simulink model "Template_v4_1_0_2024b_Jetson"  (R2024b)
settings: Solver=ode4  StartTime=0.0  StopTime=tsim  FixedStep=baseRate  RelTol=1e-6  AbsTol=1e-6
undefined symbols (not defined in the file): a1, a2, a3, b0, b1, b2, b3, baseRate, dataRate, DiscIntNeverNeededParam, drop_states_ARM, drop_states_BLACK, drop_states_BLUE, drop_states_RED, F_black_X_nominal, F_black_Y_nominal, F_blue_X_nominal, F_blue_Y_nominal, F_red_X_nominal, F_red_Y_nominal, F_thrusters_BLACK, F_thrusters_BLUE, F_thrusters_RED, Gamma1_el, Gamma1_sh, Gamma1_wr, Gamma2_el, Gamma2_sh, Gamma2_wr, Gamma3_el, Gamma3_sh, Gamma3_wr, Gamma4_el, Gamma4_sh, Gamma4_wr, Gamma5_el, Gamma5_sh, Gamma5_wr, Gamma6_el, Gamma6_sh, Gamma6_wr, home_states_BLACK, home_states_BLUE, home_states_RED, IBLACK, IBLUE, IDIST, IEE, init_states_BLACK, init_states_BLUE, init_states_RED, IPROX, IRED, K_BLACK, K_BLUE, K_RED, Kd_elarm, Kd_sharm, Kd_tb, Kd_tblue ... (+49)
libraries: simulink x30, dspsigops x12, nvidiaSharedBlocks x12, MainLibrary x5, dspinverses x3, nvidiaIMUSensorslib x1
(part 3 of 7)

== system Template_v4_1_0_2024b_Jetson/Gyro.//Accel. Code/Log Gyro//Accel ==
  Action Port : ActionPort  ActionPortLabel=if(u1 == 0)
  Data Store Read : DataStoreRead  DataStoreName=WhoAmI  IndexOptions=Index vector (dialog)  Indices=1  OutputSizes=1
  Data Store Write10 : DataStoreWrite  DataStoreName=BLACK_IMU_Measurements  IndexOptions=Index vector (dialog)  Indices=1  OutputSizes=1
  Data Store Write11 : DataStoreWrite  DataStoreName=BLUE_IMU_Measurements  IndexOptions=Index vector (dialog)  Indices=1  OutputSizes=1
  Data Store Write9 : DataStoreWrite  DataStoreName=RED_IMU_Measurements  IndexOptions=Index vector (dialog)  Indices=1  OutputSizes=1
  Demux : Demux  Outputs=3
  Demux1 : Demux  Outputs=3
  Gyroscope/Accelerometer : nvidiaIMUSensorslib/BMI160  I2CModule=1  I2CAddress=0x69  EnableSecondaryMag=on  MagnetometerI2CAddress=0x10  BitRate=1000000  IsActiveAccel=on  IsActiveGyro=on  IsActiveMag=off  IsActiveTemperature=off  IsIntSource=off  IsTapEventSource=off  IsHighGEventSource=off  IsAnyMotionEventSource=off  IsAccelStatus=off  IsGyroStatus=off  IsMagStatus=off  AccelerationRange=+/- 2g  AccelerometerODR=100 Hz  IsEnableAccelLowPassFilter=off  AccelerometerFilterMode=Normal  GyroscopeRange=125 dps  GyroscopeODR=100 Hz  IsEnableGyroLowPassFilter=off  GyroscopeFilterMode=Normal  MagnetometerODR=25 Hz  IsSingleTap=off  SingleTapQuietTimeThreshold=30 ms  SingleTapShockTimeThreshold=50 ms  SingleTapAmplitudeThreshold2g=0.1  SingleTapAmplitudeThreshold4g=0.1  SingleTapAmplitudeThreshold8g=0.2  SingleTapAmplitudeThreshold16g=0.3  InterruptPinSingleTap=INT1  IsDoubleTap=off  DoubleTapDurationTimeThreshold=50 ms  InterruptPinDoubleTap=INT1  IsHighGDetection=off  HighGTimeThreshold=2.5  HighGAmplitudeThreshold2g=0.1  HighGAmplitudeThreshold4g=0.1  HighGAmplitudeThreshold8g=0.1  HighGAmplitudeThreshold16g=0.1  InterruptPinHighG=INT1  IsAnyMotion=off  AnyMotionTimeThreshold=1  AnyMotionAmplitudeThreshold2g=0.1  AnyMotionAmplitudeThreshold4g=0.1  AnyMotionAmplitudeThreshold8g=0.1  AnyMotionAmplitudeThreshold16g=0.1  InterruptPinAnyMotion=INT1  IsSlowMotion=off  SlowMotionTimeThreshold=1  SlowMotionAmplitudeThreshold2g=0.1  SlowMotionAmplitudeThreshold4g=0.1  SlowMotionAmplitudeThreshold8g=0.1  SlowMotionAmplitudeThreshold16g=0.1  InterruptPinSlowMotion=INT1  IsFlatDetection=off  FlatThetaThreshold=5  FlatTimeThreshold=640 ms  InterruptPinFlat=INT1  IsDataReady=off  InterruptPinDataReady=INT1  IsFifo=off  FifoMode=Full Buffer  InterruptPinFifo=INT1  DataType=double  SampleTime=-1
  Mux : Mux  Inputs=3
  Mux1 : Mux  Inputs=3
  Mux2 : Mux  Inputs=3
  Parse IMU Data : MATLAB Function  TreatAsAtomicUnit=on
  Terminator : Terminator
  Terminator1 : Terminator
  Terminator2 : Terminator
  wires:
  Demux1/3 -> Parse IMU Data/4(IMU_Gz)
  Gyroscope/Accelerometer/1 -> Demux/1
  Demux1/1 -> Terminator1/1
  Parse IMU Data/4(BLACK_IMU_Ax) -> Mux1/1
  Parse IMU Data/1(RED_IMU_Ax) -> Mux/1
  Parse IMU Data/8(BLUE_IMU_Ay) -> Mux2/2
  Parse IMU Data/3(RED_IMU_Gz) -> Mux/3
  Demux/3 -> Terminator/1
  Parse IMU Data/6(BLACK_IMU_Gz) -> Mux1/3
  Parse IMU Data/5(BLACK_IMU_Ay) -> Mux1/2
  Demux1/2 -> Terminator2/1
  Parse IMU Data/9(BLUE_IMU_Gz) -> Mux2/3
  Gyroscope/Accelerometer/2 -> Demux1/1
  Parse IMU Data/2(RED_IMU_Ay) -> Mux/2
  Parse IMU Data/7(BLUE_IMU_Ax) -> Mux2/1
  Demux/2 -> Parse IMU Data/3(IMU_Ay)
  Data Store Read/1 -> Parse IMU Data/1(WhoAmI)
  Demux/1 -> Parse IMU Data/2(IMU_Ax)
  Mux/1 -> Data Store Write9/1
  Mux1/1 -> Data Store Write10/1
  Mux2/1 -> Data Store Write11/1

== system Template_v4_1_0_2024b_Jetson/Manipulator Encoder Data/Change ARM Behavior ==
  Action Port : ActionPort  ActionPortLabel=if(u1 == 1 & u2 == 0)
  Data Store Write : DataStoreWrite  DataStoreName=ARM_Measured_States  IndexOptions=Index vector (dialog)  Indices=1  OutputSizes=1
  Delay : Delay  DelayLength=1
  Delay1 : Delay  DelayLength=1
  Delay2 : Delay  DelayLength=1
  Mux : Mux  Inputs=6
  Read Joint Positions using Dynamixel Encoders : MainLibrary/Dynamixel Functions/Read Joint Positions using  Dynamixel Encoders  SampleTime=baseRate
      settings: SourceProductName=SPOT Custom Library
  wires:
  Delay/1 -> Read Joint Positions using Dynamixel Encoders/1
  Read Joint Positions using Dynamixel Encoders/5 -> Mux/5
  Read Joint Positions using Dynamixel Encoders/6 -> Mux/6
  Delay1/1 -> Read Joint Positions using Dynamixel Encoders/2
  Read Joint Positions using Dynamixel Encoders/2 -> Mux/2, Delay1/1
  Delay2/1 -> Read Joint Positions using Dynamixel Encoders/3
  Read Joint Positions using Dynamixel Encoders/1 -> Mux/1, Delay/1
  Read Joint Positions using Dynamixel Encoders/3 -> Mux/3, Delay2/1
  Read Joint Positions using Dynamixel Encoders/4 -> Mux/4
  Mux/1 -> Data Store Write/1

== system Template_v4_1_0_2024b_Jetson/PhaseSpace Camera Code/Initialize Universal Time (Simulation) ==
  Action Port : ActionPort  ActionPortLabel=elseif(u1 == 1)
  Set Universal Time (If this is a simulation) : Clock
  Universal_Time : DataStoreWrite  DataStoreName=Univ_Time  IndexOptions=Index vector (dialog)  Indices=1  OutputSizes=1
  wires:
  Set Universal Time (If this is a simulation)/1 -> Universal_Time/1

== system Template_v4_1_0_2024b_Jetson/PhaseSpace Camera Code/Use Hardware to Obtain States ==
  Action Port : ActionPort  ActionPortLabel=if(u1 == 0)
  Demux : Demux  Outputs=[4,3,3,9]
  Demux1 : Demux  Outputs=[3,3,3]
  Receive and Process Phasespace Data : Subsystem
  Store BLACK Data : Subsystem
  Store BLUE Data : Subsystem
  Store RED Data : Subsystem
  wires:
  Receive and Process Phasespace Data/1(PhaseSpace Data) -> Demux/1
  Demux/1 -> Store RED Data/1(RED Data)
  Demux/2 -> Store BLACK Data/1(BLACK Data)
  Demux/3 -> Store BLUE Data/1(BLUE Data)
  Demux/4 -> Demux1/1
  Demux1/1 -> Store RED Data/2(RED Velocities)
  Demux1/2 -> Store BLACK Data/2(BLACK Velocities)
  Demux1/3 -> Store BLUE Data/2(BLUE Velocities)
  Receive and Process Phasespace Data/2(PhaseSpace Clock) -> Store RED Data/3(PS Clock), Store BLACK Data/3(PS Clock), Store BLUE Data/3(PS Clock)

== system Template_v4_1_0_2024b_Jetson/Platform Identification/Subsystem ==
  Action Port : ActionPort  ActionPortLabel=if(u1 == 0)
  Data Store Write : DataStoreWrite  DataStoreName=WhoAmI  IndexOptions=Index vector (dialog)  Indices=1  OutputSizes=1
  WhoAmI : MainLibrary/WhoAmI  SampleTime=baseRate
      settings: SourceProductName=SPOT Custom Library
  wires:
  WhoAmI/1 -> Data Store Write/1

== system Template_v4_1_0_2024b_Jetson/Robotic Arm Code/Change ARM Behavior ==
  Action Port : ActionPort  ActionPortLabel=if(u1 == 1 & u2 == 0)
  Arm Control Mode : DataStoreRead  DataStoreName=ARM_Control_Mode  IndexOptions=Index vector (dialog)  Indices=1  OutputSizes=1
  Command : DataStoreRead  DataStoreName=ARM_Controls  IndexOptions=Index vector (dialog)  Indices=1  OutputSizes=1
  "Control Dynamixel Actuators in either Position, Current, or Speed Control Modes" : MainLibrary/Dynamixel Functions/Control Dynamixel Actuators in  either Position, Current, or Speed  Control Modes  POSITION_P_GAIN=400  POSITION_I_GAIN=0  POSITION_D_GAIN=200  MAX_POSITION=3072  MIN_POSITION=1024  MOVE_TIME=0  CURRENT_LIMIT=850  SPEED_P_GAIN=400  SPEED_I_GAIN=100  VELOCITY_LIMIT=50  ACCELERATION_TIME=0  SampleTime=baseRate
      settings: SourceProductName=SPOT Custom Library
  Demux : Demux  Outputs=3
  wires:
  Arm Control Mode/1 -> "Control Dynamixel Actuators in either Position, Current, or Speed Control Modes"/1
  Command/1 -> Demux/1
  Demux/1 -> "Control Dynamixel Actuators in either Position, Current, or Speed Control Modes"/2
  Demux/2 -> "Control Dynamixel Actuators in either Position, Current, or Speed Control Modes"/3
  Demux/3 -> "Control Dynamixel Actuators in either Position, Current, or Speed Control Modes"/4

== system Template_v4_1_0_2024b_Jetson/Send Data to Orin/Subsystem ==
  Action Port : ActionPort  ActionPortLabel=if(u1 == 0)
  BLACK States : DataStoreRead  DataStoreName=BLACK_Measured_States  IndexOptions=Index vector (dialog)  Indices=1  OutputSizes=1
  BLUE States : DataStoreRead  DataStoreName=BLUE_Measured_States  IndexOptions=Index vector (dialog)  Indices=1  OutputSizes=1
  Mux : Mux
  RED States : DataStoreRead  DataStoreName=RED_Measured_States  IndexOptions=Index vector (dialog)  Indices=1  OutputSizes=1
  Time : DataStoreRead  DataStoreName=Univ_Time  IndexOptions=Index vector (dialog)  Indices=1  OutputSizes=1
  UDP Send : nvidiaSharedBlocks/UDP Send  remoteURL='192.168.1.115'  remotePort=46875  localURL='0.0.0.0'  localPortSource=Automatically determine  localPort=-1  sampletime=-1  blockPlatform=NVIDIA  separateLengthPort=0
      settings: LibrarySourceBlock=nvidiaNetworklib/UDP Send
  wires:
  Mux/1 -> UDP Send/1
  Time/1 -> Mux/1
  RED States/1 -> Mux/2
  BLACK States/1 -> Mux/3
  BLUE States/1 -> Mux/4

== system Template_v4_1_0_2024b_Jetson/Simulate Plant Dynamics/BLACK Dynamics ==
  Add Noise : RandomNumber  Variance=1e-9  SampleTime=baseRate
  Calculated & Store Measured States : Subsystem
  Calculated & Store True States : Subsystem
  Data @ Measurement Rate : Subsystem
  Dynamics Model for BLACK : Subsystem  SystemSampleTime=serverRate
      settings: PortSchema="{\"entries\":[{\"content\":{\"sides\":[{\"content\":{\"connectorIds\":[\"In1\"]},\"type\":\"ConnectorPlacement.EquallySpacedRectSide\",\"uuid\":\"9df3cfb7-f920-4c45-b004-2d63eab5f007\"},{\"content\":{\"side\":\"RIGHT\"},\"type\":\"ConnectorPlacement.EquallySpacedRectSide\",\"uuid\":\"24f4b70f-864f-4cab-bc2b-b450467a01b3\"},{\"content\":{\"connectorIds\":[\"Out1\"],\"side\":\"TOP\"},\"type\":\"ConnectorPlacement.EquallySpacedRectSide\",\"uuid\":\"64c0236c-f70a-4099-950e-ee3e8643e7f2\"}]},\"type\":\"ConnectorPlacement.EquallySpacedConnector\",\"uuid\":\"dd7c693a-185b-4c5f-873e-b9df56bea395\"}],\"packageUris\":[\"http://schema.mathworks.com/mf0/Connector/R2020b\"],\"version\":\"1.0\"}"
  Saturated Control Commands for BLACK : DataStoreRead  DataStoreName=BLACK_Saturated_Controls  IndexOptions=Index vector (dialog)  Indices=1  OutputSizes=1
  Sum : Sum  Inputs=++|
  wires:
  Dynamics Model for BLACK/1(states) -> Sum/2, Calculated & Store True States/1(y)
  Data @ Measurement Rate/2(Time Step) -> Calculated & Store Measured States/2(dt)
  Saturated Control Commands for BLACK/1 -> Dynamics Model for BLACK/1(control_inputs)
  Data @ Measurement Rate/1(Data Held) -> Calculated & Store Measured States/1(y)
  Sum/1 -> Data @ Measurement Rate/1(Data Input)
  Add Noise/1 -> Sum/1

== system Template_v4_1_0_2024b_Jetson/Simulate Plant Dynamics/BLUE Dynamics ==
  Add Noise : RandomNumber  Variance=1e-9  SampleTime=baseRate
  BLUE  Dynamics Model : Subsystem  SystemSampleTime=serverRate
      settings: PortSchema="{\"entries\":[{\"content\":{\"sides\":[{\"content\":{\"connectorIds\":[\"In1\"]},\"type\":\"ConnectorPlacement.EquallySpacedRectSide\",\"uuid\":\"9df3cfb7-f920-4c45-b004-2d63eab5f007\"},{\"content\":{\"side\":\"RIGHT\"},\"type\":\"ConnectorPlacement.EquallySpacedRectSide\",\"uuid\":\"24f4b70f-864f-4cab-bc2b-b450467a01b3\"},{\"content\":{\"connectorIds\":[\"Out1\"],\"side\":\"TOP\"},\"type\":\"ConnectorPlacement.EquallySpacedRectSide\",\"uuid\":\"64c0236c-f70a-4099-950e-ee3e8643e7f2\"}]},\"type\":\"ConnectorPlacement.EquallySpacedConnector\",\"uuid\":\"dd7c693a-185b-4c5f-873e-b9df56bea395\"}],\"packageUris\":[\"http://schema.mathworks.com/mf0/Connector/R2020b\"],\"version\":\"1.0\"}"
  Calculated & Store Measured States : Subsystem
  Calculated & Store True States : Subsystem
  Data @ Measurement Rate : Subsystem
  Saturated Control Commands for BLUE : DataStoreRead  DataStoreName=BLUE_Saturated_Controls  IndexOptions=Index vector (dialog)  Indices=1  OutputSizes=1
  Sum1 : Sum  Inputs=++|
  wires:
  Saturated Control Commands for BLUE/1 -> BLUE  Dynamics Model/1(control_inputs)
  Data @ Measurement Rate/2(Time Step) -> Calculated & Store Measured States/2(dt)
  Add Noise/1 -> Sum1/1
  BLUE  Dynamics Model/1(states) -> Sum1/2, Calculated & Store True States/1(y)
  Sum1/1 -> Data @ Measurement Rate/1(Data Input)
  Data @ Measurement Rate/1(Data Held) -> Calculated & Store Measured States/1(y)

== system Template_v4_1_0_2024b_Jetson/Simulate Plant Dynamics/RED and ARM Dynamics ==
  Constant : Constant  Value=platformSelection
  If : If  IfExpression=u1 == 4 | u1 == 5 | u1 == 10 | u1 == 11
  RED + ARM : Subsystem  TreatAsAtomicUnit=on
  RED Only : Subsystem  TreatAsAtomicUnit=on
  wires:
  If/1 -> RED + ARM/Action
  Constant/1 -> If/1
  If/2 -> RED Only/Action

== system Template_v4_1_0_2024b_Jetson/Thruster Control Code/Change BLACK Behavior ==
  note: Calculate the percentage of time each thruster must be on, and send to the PWM blocks.
  note: Using the attitude, rotate the forces into the body frame.
  note: Calculate which thrusters must be turned on and for how long.
  Action Port : ActionPort  ActionPortLabel=if(u1 == 2 | u2 == 1)
  BLACK Controls : DataStoreRead  DataStoreName=BLACK_Controls  IndexOptions=Index vector (dialog)  Indices=1  OutputSizes=1
  BLACK States : DataStoreRead  DataStoreName=BLACK_Measured_States  IndexOptions=Index vector (dialog)  Indices=1  OutputSizes=1
  Calculate Duty Cycle : Subsystem
  Data Store Write2 : DataStoreWrite  DataStoreName=BLACK_Saturated_Controls  IndexOptions=Index vector (dialog)  Indices=1  OutputSizes=1
  Demux1 : Demux  Outputs=[2,1]
  Demux2 : Demux  Outputs=[2,1,6]
  Mux : Mux  Inputs=2
  Rotate Forces to Body : Subsystem
  Terminator : Terminator
  Terminator1 : Terminator
  BLACK DC : Outport  VectorParamsAs1DForOutWhenUnconnected=off
  wires:
  Calculate Duty Cycle/2(Saturated Forces Moments) -> Data Store Write2/1
  Rotate Forces to Body/1(F_b) -> Mux/1
  Demux1/2 -> Mux/2
  Calculate Duty Cycle/1(Duty Cycle) -> BLACK DC/1
  Mux/1 -> Calculate Duty Cycle/1("[Fx_b; Fy_b; Tz]")
  BLACK Controls/1 -> Demux1/1
  Demux1/1 -> Rotate Forces to Body/1("F_I ")
  BLACK States/1 -> Demux2/1
  Demux2/1 -> Terminator/1
  Demux2/3 -> Terminator1/1
  Demux2/2 -> Calculate Duty Cycle/2(Measured Attitude), Rotate Forces to Body/2(Rz)

== system Template_v4_1_0_2024b_Jetson/Thruster Control Code/Change BLUE Behavior ==
  note: Calculate the percentage of time each thruster must be on, and send to the PWM blocks.
  note: Using the attitude, rotate the forces into the body frame.
  note: Calculate which thrusters must be turned on and for how long.
  Action Port : ActionPort  ActionPortLabel=if(u1 == 3 | u2 == 1)
  Calculate Duty Cycle : Subsystem
  Data Store Read : DataStoreRead  DataStoreName=BLUE_Controls  IndexOptions=Index vector (dialog)  Indices=1  OutputSizes=1
  Data Store Read1 : DataStoreRead  DataStoreName=BLUE_Measured_States  IndexOptions=Index vector (dialog)  Indices=1  OutputSizes=1
  Data Store Write3 : DataStoreWrite  DataStoreName=BLUE_Saturated_Controls  IndexOptions=Index vector (dialog)  Indices=1  OutputSizes=1
  Demux : Demux  Outputs=[2,1]
  Demux1 : Demux  Outputs=[2,1,6]
  Mux1 : Mux  Inputs=2
  Rotate Forces to Body : Subsystem
  Terminator : Terminator
  Terminator1 : Terminator
  BLUE DC : Outport  VectorParamsAs1DForOutWhenUnconnected=off
  wires:
  Calculate Duty Cycle/1(Duty Cycle) -> BLUE DC/1
  Rotate Forces to Body/1(F_b) -> Mux1/1
  Demux/2 -> Mux1/2
  Mux1/1 -> Calculate Duty Cycle/1("[Fx_b; Fy_b; Tz]")
  Calculate Duty Cycle/2(Saturated Forces Moments) -> Data Store Write3/1
  Data Store Read/1 -> Demux/1
  Demux/1 -> Rotate Forces to Body/1("F_I ")
  Data Store Read1/1 -> Demux1/1
  Demux1/2 -> Calculate Duty Cycle/2(Measured Attitude), Rotate Forces to Body/2(Rz)
  Demux1/1 -> Terminator/1
  Demux1/3 -> Terminator1/1

== system Template_v4_1_0_2024b_Jetson/Thruster Control Code/Change RED Behavior ==
  note: Calculate which thrusters must be turned on and for how long.
  note: Calculate the percentage of time each thruster must be on, and send to the PWM blocks.
  note: Using the attitude, rotate the forces into the body frame.
  Action Port : ActionPort  ActionPortLabel=if(u1 == 1 | u2 == 1)
  Calculate Duty Cycle : Subsystem
  Data Store Read : DataStoreRead  DataStoreName=RED_Controls  IndexOptions=Index vector (dialog)  Indices=1  OutputSizes=1
  Data Store Read1 : DataStoreRead  DataStoreName=RED_Measured_States  IndexOptions=Index vector (dialog)  Indices=1  OutputSizes=1
  Data Store Write3 : DataStoreWrite  DataStoreName=RED_Saturated_Controls  IndexOptions=Index vector (dialog)  Indices=1  OutputSizes=1
  Demux : Demux  Outputs=[2,1]
  Demux1 : Demux  Outputs=[2,1,6]
  Mux1 : Mux  Inputs=2
  Rotate Forces to Body : Subsystem
  Terminator : Terminator
  Terminator1 : Terminator
  RED DC : Outport  VectorParamsAs1DForOutWhenUnconnected=off
  wires:
  Calculate Duty Cycle/2(Saturated Forces Moments) -> Data Store Write3/1
  Demux/1 -> Rotate Forces to Body/1("F_I ")
  Mux1/1 -> Calculate Duty Cycle/1("[Fx_b; Fy_b; Tz]")
  Demux/2 -> Mux1/2
  Demux1/2 -> Calculate Duty Cycle/2(Measured Attitude), Rotate Forces to Body/2(Rz)
  Rotate Forces to Body/1(F_b) -> Mux1/1
  Calculate Duty Cycle/1(Duty Cycle) -> RED DC/1
  Data Store Read/1 -> Demux/1
  Demux1/1 -> Terminator/1
  Demux1/3 -> Terminator1/1
  Data Store Read1/1 -> Demux1/1

== system Template_v4_1_0_2024b_Jetson/1 - Experiment Logic/Phase #2: Initial Position/Desired Joint Angles RED ==
  Constant1 : Constant  Value=pi/2
  Constant2 : Constant  Value=0
  Constant3 : Constant  Value=pi/2
  Mux : Mux  Inputs=3
  Target Array : Outport
  wires:
  Mux/1 -> Target Array/1
  Constant3/1 -> Mux/1
  Constant1/1 -> Mux/2
  Constant2/1 -> Mux/3

== system Template_v4_1_0_2024b_Jetson/1 - Experiment Logic/Phase #2: Initial Position/Desired Position BLACK ==
  Desired States (BLACK) : Constant  Value=init_states_BLACK  SampleTime=-1
  Target Array : Outport
  wires:
  Desired States (BLACK)/1 -> Target Array/1

== system Template_v4_1_0_2024b_Jetson/1 - Experiment Logic/Phase #2: Initial Position/Desired Position BLUE ==
  Desired States (BLUE) : Constant  Value=init_states_BLUE  SampleTime=-1
  Target Array : Outport
  wires:
  Desired States (BLUE)/1 -> Target Array/1

== system Template_v4_1_0_2024b_Jetson/1 - Experiment Logic/Phase #2: Initial Position/Desired Position RED ==
  Constant2 : Constant  Value=init_states_RED
  Target Array : Outport
  wires:
  Constant2/1 -> Target Array/1

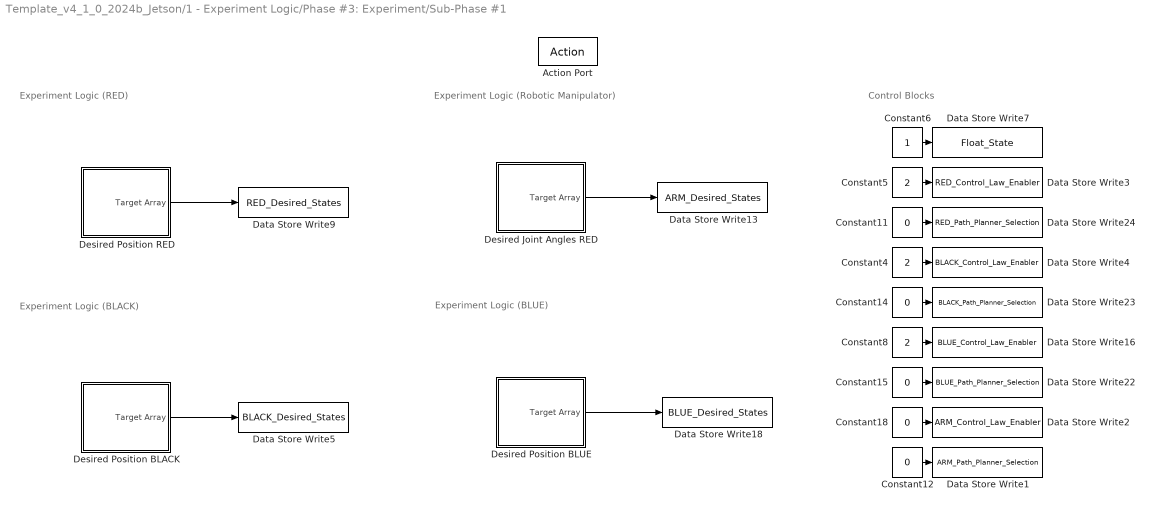
== system Template_v4_1_0_2024b_Jetson/1 - Experiment Logic/Phase #3: Experiment/Sub-Phase #1 ==
  note: Experiment Logic (BLUE)
  note: Experiment Logic (Robotic Manipulator)
  note: Experiment Logic (RED)
  note: Experiment Logic (BLACK)
  note: Control Blocks
  Action Port : ActionPort  ActionPortLabel=if(u1 < u2)
  Constant{11..12,14..15,18} (5 alike) : Constant  Value=0
  Constant4 : Constant  Value=2
  Constant5 : Constant  Value=2
  Constant6 : Constant
  Constant8 : Constant  Value=2
  Data Store Write1 : DataStoreWrite  DataStoreName=ARM_Path_Planner_Selection  IndexOptions=Index vector (dialog)  Indices=1  OutputSizes=1
  Data Store Write13 : DataStoreWrite  DataStoreName=ARM_Desired_States  IndexOptions=Index vector (dialog)  Indices=1  OutputSizes=1
  Data Store Write16 : DataStoreWrite  DataStoreName=BLUE_Control_Law_Enabler  IndexOptions=Index vector (dialog)  Indices=1  OutputSizes=1
  Data Store Write18 : DataStoreWrite  DataStoreName=BLUE_Desired_States  IndexOptions=Index vector (dialog)  Indices=1  OutputSizes=1
  Data Store Write2 : DataStoreWrite  DataStoreName=ARM_Control_Law_Enabler  IndexOptions=Index vector (dialog)  Indices=1  OutputSizes=1
  Data Store Write22 : DataStoreWrite  DataStoreName=BLUE_Path_Planner_Selection  IndexOptions=Index vector (dialog)  Indices=1  OutputSizes=1
  Data Store Write23 : DataStoreWrite  DataStoreName=BLACK_Path_Planner_Selection  IndexOptions=Index vector (dialog)  Indices=1  OutputSizes=1
  Data Store Write24 : DataStoreWrite  DataStoreName=RED_Path_Planner_Selection  IndexOptions=Index vector (dialog)  Indices=1  OutputSizes=1
  Data Store Write3 : DataStoreWrite  DataStoreName=RED_Control_Law_Enabler  IndexOptions=Index vector (dialog)  Indices=1  OutputSizes=1
  Data Store Write4 : DataStoreWrite  DataStoreName=BLACK_Control_Law_Enabler  IndexOptions=Index vector (dialog)  Indices=1  OutputSizes=1
  Data Store Write5 : DataStoreWrite  DataStoreName=BLACK_Desired_States  IndexOptions=Index vector (dialog)  Indices=1  OutputSizes=1
  Data Store Write7 : DataStoreWrite  DataStoreName=Float_State  IndexOptions=Index vector (dialog)  Indices=1  OutputSizes=1
  Data Store Write9 : DataStoreWrite  DataStoreName=RED_Desired_States  IndexOptions=Index vector (dialog)  Indices=1  OutputSizes=1
  Desired Joint Angles RED : Subsystem
  Desired Position BLACK : Subsystem
  Desired Position BLUE : Subsystem
  Desired Position RED : Subsystem
  wires:
  Desired Position BLACK/1(Target Array) -> Data Store Write5/1
  Desired Position BLUE/1(Target Array) -> Data Store Write18/1
  Desired Position RED/1(Target Array) -> Data Store Write9/1
  Desired Joint Angles RED/1(Target Array) -> Data Store Write13/1
  Constant12/1 -> Data Store Write1/1
  Constant18/1 -> Data Store Write2/1
  Constant6/1 -> Data Store Write7/1
  Constant15/1 -> Data Store Write22/1
  Constant14/1 -> Data Store Write23/1
  Constant5/1 -> Data Store Write3/1
  Constant11/1 -> Data Store Write24/1
  Constant8/1 -> Data Store Write16/1
  Constant4/1 -> Data Store Write4/1

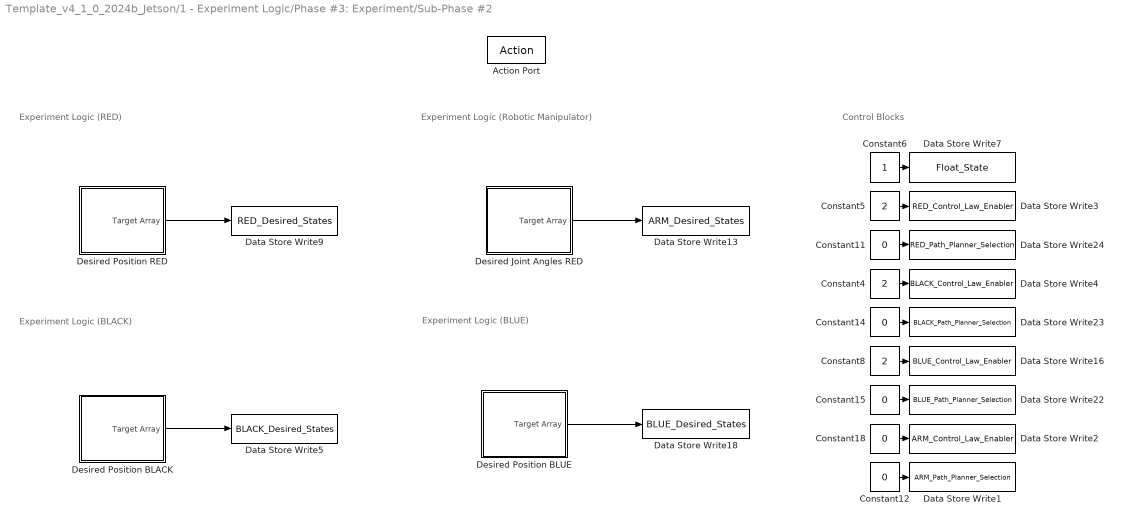
== system Template_v4_1_0_2024b_Jetson/1 - Experiment Logic/Phase #3: Experiment/Sub-Phase #2  ==
  note: Experiment Logic (BLACK)
  note: Experiment Logic (Robotic Manipulator)
  note: Experiment Logic (BLUE)
  note: Experiment Logic (RED)
  note: Control Blocks
  Action Port : ActionPort  ActionPortLabel=elseif((u1 < u3 & u1 >= u2))
  Constant{11..12,14..15,18} (5 alike) : Constant  Value=0
  Constant4 : Constant  Value=2
  Constant5 : Constant  Value=2
  Constant6 : Constant
  Constant8 : Constant  Value=2
  Data Store Write1 : DataStoreWrite  DataStoreName=ARM_Path_Planner_Selection  IndexOptions=Index vector (dialog)  Indices=1  OutputSizes=1
  Data Store Write13 : DataStoreWrite  DataStoreName=ARM_Desired_States  IndexOptions=Index vector (dialog)  Indices=1  OutputSizes=1
  Data Store Write16 : DataStoreWrite  DataStoreName=BLUE_Control_Law_Enabler  IndexOptions=Index vector (dialog)  Indices=1  OutputSizes=1
  Data Store Write18 : DataStoreWrite  DataStoreName=BLUE_Desired_States  IndexOptions=Index vector (dialog)  Indices=1  OutputSizes=1
  Data Store Write2 : DataStoreWrite  DataStoreName=ARM_Control_Law_Enabler  IndexOptions=Index vector (dialog)  Indices=1  OutputSizes=1
  Data Store Write22 : DataStoreWrite  DataStoreName=BLUE_Path_Planner_Selection  IndexOptions=Index vector (dialog)  Indices=1  OutputSizes=1
  Data Store Write23 : DataStoreWrite  DataStoreName=BLACK_Path_Planner_Selection  IndexOptions=Index vector (dialog)  Indices=1  OutputSizes=1
  Data Store Write24 : DataStoreWrite  DataStoreName=RED_Path_Planner_Selection  IndexOptions=Index vector (dialog)  Indices=1  OutputSizes=1
  Data Store Write3 : DataStoreWrite  DataStoreName=RED_Control_Law_Enabler  IndexOptions=Index vector (dialog)  Indices=1  OutputSizes=1
  Data Store Write4 : DataStoreWrite  DataStoreName=BLACK_Control_Law_Enabler  IndexOptions=Index vector (dialog)  Indices=1  OutputSizes=1
  Data Store Write5 : DataStoreWrite  DataStoreName=BLACK_Desired_States  IndexOptions=Index vector (dialog)  Indices=1  OutputSizes=1
  Data Store Write7 : DataStoreWrite  DataStoreName=Float_State  IndexOptions=Index vector (dialog)  Indices=1  OutputSizes=1
  Data Store Write9 : DataStoreWrite  DataStoreName=RED_Desired_States  IndexOptions=Index vector (dialog)  Indices=1  OutputSizes=1
  Desired Joint Angles RED : Subsystem
  Desired Position BLACK : Subsystem
  Desired Position BLUE : Subsystem
  Desired Position RED : Subsystem
  wires:
  Desired Position RED/1(Target Array) -> Data Store Write9/1
  Desired Position BLACK/1(Target Array) -> Data Store Write5/1
  Desired Position BLUE/1(Target Array) -> Data Store Write18/1
  Constant12/1 -> Data Store Write1/1
  Constant18/1 -> Data Store Write2/1
  Constant6/1 -> Data Store Write7/1
  Constant15/1 -> Data Store Write22/1
  Constant14/1 -> Data Store Write23/1
  Constant5/1 -> Data Store Write3/1
  Constant11/1 -> Data Store Write24/1
  Constant8/1 -> Data Store Write16/1
  Constant4/1 -> Data Store Write4/1
  Desired Joint Angles RED/1(Target Array) -> Data Store Write13/1

== system Template_v4_1_0_2024b_Jetson/1 - Experiment Logic/Phase #3: Experiment/Sub-Phase #3  ==
  note: Experiment Logic (BLACK)
  note: Experiment Logic (Robotic Manipulator)
  note: Experiment Logic (BLUE)
  note: Experiment Logic (RED)
  note: Control Blocks
  Action Port : ActionPort  ActionPortLabel=elseif((u1 < u4 & u1 >= u3))
  Constant{11..12,14..15,18} (5 alike) : Constant  Value=0
  Constant4 : Constant  Value=2
  Constant5 : Constant  Value=2
  Constant6 : Constant
  Constant8 : Constant  Value=2
  Data Store Write1 : DataStoreWrite  DataStoreName=ARM_Path_Planner_Selection  IndexOptions=Index vector (dialog)  Indices=1  OutputSizes=1
  Data Store Write13 : DataStoreWrite  DataStoreName=ARM_Desired_States  IndexOptions=Index vector (dialog)  Indices=1  OutputSizes=1
  Data Store Write16 : DataStoreWrite  DataStoreName=BLUE_Control_Law_Enabler  IndexOptions=Index vector (dialog)  Indices=1  OutputSizes=1
  Data Store Write18 : DataStoreWrite  DataStoreName=BLUE_Desired_States  IndexOptions=Index vector (dialog)  Indices=1  OutputSizes=1
  Data Store Write2 : DataStoreWrite  DataStoreName=ARM_Control_Law_Enabler  IndexOptions=Index vector (dialog)  Indices=1  OutputSizes=1
  Data Store Write22 : DataStoreWrite  DataStoreName=BLUE_Path_Planner_Selection  IndexOptions=Index vector (dialog)  Indices=1  OutputSizes=1
  Data Store Write23 : DataStoreWrite  DataStoreName=BLACK_Path_Planner_Selection  IndexOptions=Index vector (dialog)  Indices=1  OutputSizes=1
  Data Store Write24 : DataStoreWrite  DataStoreName=RED_Path_Planner_Selection  IndexOptions=Index vector (dialog)  Indices=1  OutputSizes=1
  Data Store Write3 : DataStoreWrite  DataStoreName=RED_Control_Law_Enabler  IndexOptions=Index vector (dialog)  Indices=1  OutputSizes=1
  Data Store Write4 : DataStoreWrite  DataStoreName=BLACK_Control_Law_Enabler  IndexOptions=Index vector (dialog)  Indices=1  OutputSizes=1
  Data Store Write5 : DataStoreWrite  DataStoreName=BLACK_Desired_States  IndexOptions=Index vector (dialog)  Indices=1  OutputSizes=1
  Data Store Write7 : DataStoreWrite  DataStoreName=Float_State  IndexOptions=Index vector (dialog)  Indices=1  OutputSizes=1
  Data Store Write9 : DataStoreWrite  DataStoreName=RED_Desired_States  IndexOptions=Index vector (dialog)  Indices=1  OutputSizes=1
  Desired Joint Angles RED : Subsystem
  Desired Position BLACK : Subsystem
  Desired Position BLUE : Subsystem
  Desired Position RED : Subsystem
  wires:
  Desired Position RED/1(Target Array) -> Data Store Write9/1
  Desired Position BLACK/1(Target Array) -> Data Store Write5/1
  Desired Position BLUE/1(Target Array) -> Data Store Write18/1
  Desired Joint Angles RED/1(Target Array) -> Data Store Write13/1
  Constant12/1 -> Data Store Write1/1
  Constant18/1 -> Data Store Write2/1
  Constant6/1 -> Data Store Write7/1
  Constant15/1 -> Data Store Write22/1
  Constant14/1 -> Data Store Write23/1
  Constant5/1 -> Data Store Write3/1
  Constant11/1 -> Data Store Write24/1
  Constant8/1 -> Data Store Write16/1
  Constant4/1 -> Data Store Write4/1

== system Template_v4_1_0_2024b_Jetson/1 - Experiment Logic/Phase #3: Experiment/Sub-Phase #4 ==
  note: Experiment Logic (BLACK)
  note: Experiment Logic (Robotic Manipulator)
  note: Experiment Logic (BLUE)
  note: Experiment Logic (RED)
  note: Control Blocks
  Action Port : ActionPort  ActionPortLabel=elseif( (u1 < u5 & u1 >= u4))
  Constant{11..12,14..15,18} (5 alike) : Constant  Value=0
  Constant4 : Constant  Value=2
  Constant5 : Constant  Value=2
  Constant6 : Constant
  Constant8 : Constant  Value=2
  Data Store Write1 : DataStoreWrite  DataStoreName=ARM_Path_Planner_Selection  IndexOptions=Index vector (dialog)  Indices=1  OutputSizes=1
  Data Store Write13 : DataStoreWrite  DataStoreName=ARM_Desired_States  IndexOptions=Index vector (dialog)  Indices=1  OutputSizes=1
  Data Store Write16 : DataStoreWrite  DataStoreName=BLUE_Control_Law_Enabler  IndexOptions=Index vector (dialog)  Indices=1  OutputSizes=1
  Data Store Write18 : DataStoreWrite  DataStoreName=BLUE_Desired_States  IndexOptions=Index vector (dialog)  Indices=1  OutputSizes=1
  Data Store Write2 : DataStoreWrite  DataStoreName=ARM_Control_Law_Enabler  IndexOptions=Index vector (dialog)  Indices=1  OutputSizes=1
  Data Store Write22 : DataStoreWrite  DataStoreName=BLUE_Path_Planner_Selection  IndexOptions=Index vector (dialog)  Indices=1  OutputSizes=1
  Data Store Write23 : DataStoreWrite  DataStoreName=BLACK_Path_Planner_Selection  IndexOptions=Index vector (dialog)  Indices=1  OutputSizes=1
  Data Store Write24 : DataStoreWrite  DataStoreName=RED_Path_Planner_Selection  IndexOptions=Index vector (dialog)  Indices=1  OutputSizes=1
  Data Store Write3 : DataStoreWrite  DataStoreName=RED_Control_Law_Enabler  IndexOptions=Index vector (dialog)  Indices=1  OutputSizes=1
  Data Store Write4 : DataStoreWrite  DataStoreName=BLACK_Control_Law_Enabler  IndexOptions=Index vector (dialog)  Indices=1  OutputSizes=1
  Data Store Write5 : DataStoreWrite  DataStoreName=BLACK_Desired_States  IndexOptions=Index vector (dialog)  Indices=1  OutputSizes=1
  Data Store Write7 : DataStoreWrite  DataStoreName=Float_State  IndexOptions=Index vector (dialog)  Indices=1  OutputSizes=1
  Data Store Write9 : DataStoreWrite  DataStoreName=RED_Desired_States  IndexOptions=Index vector (dialog)  Indices=1  OutputSizes=1
  Desired Joint Angles RED : Subsystem
  Desired Position BLACK : Subsystem
  Desired Position BLUE : Subsystem
  Desired Position RED : Subsystem
  wires:
  Desired Position RED/1(Target Array) -> Data Store Write9/1
  Desired Position BLACK/1(Target Array) -> Data Store Write5/1
  Desired Position BLUE/1(Target Array) -> Data Store Write18/1
  Desired Joint Angles RED/1(Target Array) -> Data Store Write13/1
  Constant12/1 -> Data Store Write1/1
  Constant18/1 -> Data Store Write2/1
  Constant6/1 -> Data Store Write7/1
  Constant15/1 -> Data Store Write22/1
  Constant14/1 -> Data Store Write23/1
  Constant5/1 -> Data Store Write3/1
  Constant11/1 -> Data Store Write24/1
  Constant8/1 -> Data Store Write16/1
  Constant4/1 -> Data Store Write4/1

== system Template_v4_1_0_2024b_Jetson/1 - Experiment Logic/Phase #4: Return Home/Desired Joint Angles RED ==
  Constant1 : Constant  Value=pi/2
  Constant2 : Constant  Value=0
  Constant3 : Constant  Value=pi/2
  Mux : Mux  Inputs=3
  Target Array : Outport
  wires:
  Mux/1 -> Target Array/1
  Constant3/1 -> Mux/1
  Constant1/1 -> Mux/2
  Constant2/1 -> Mux/3

== system Template_v4_1_0_2024b_Jetson/1 - Experiment Logic/Phase #4: Return Home/Desired Position BLACK ==
  Desired States (BLACK) : Constant  Value=home_states_BLACK  SampleTime=-1
  Target Array : Outport
  wires:
  Desired States (BLACK)/1 -> Target Array/1

== system Template_v4_1_0_2024b_Jetson/1 - Experiment Logic/Phase #4: Return Home/Desired Position BLUE ==
  Desired States (BLUE) : Constant  Value=home_states_BLUE  SampleTime=-1
  Target Array : Outport
  wires:
  Desired States (BLUE)/1 -> Target Array/1

== system Template_v4_1_0_2024b_Jetson/1 - Experiment Logic/Phase #4: Return Home/Desired Position RED ==
  Constant2 : Constant  Value=home_states_RED
  Target Array : Outport
  wires:
  Constant2/1 -> Target Array/1

== system Template_v4_1_0_2024b_Jetson/1 - Experiment Logic/Phase #5: Hold Home/Desired Joint Angles RED ==
  Constant1 : Constant  Value=pi/2
  Constant2 : Constant  Value=0
  Constant3 : Constant  Value=pi/2
  Mux : Mux  Inputs=3
  Target Array : Outport
  wires:
  Mux/1 -> Target Array/1
  Constant3/1 -> Mux/1
  Constant1/1 -> Mux/2
  Constant2/1 -> Mux/3

== system Template_v4_1_0_2024b_Jetson/1 - Experiment Logic/Phase #5: Hold Home/Desired Position BLACK ==
  Desired States (BLACK) : Constant  Value=home_states_BLACK  SampleTime=-1
  Target Array : Outport
  wires:
  Desired States (BLACK)/1 -> Target Array/1

== system Template_v4_1_0_2024b_Jetson/1 - Experiment Logic/Phase #5: Hold Home/Desired Position BLUE ==
  Desired States (BLUE) : Constant  Value=home_states_BLUE  SampleTime=-1
  Target Array : Outport
  wires:
  Desired States (BLUE)/1 -> Target Array/1

== system Template_v4_1_0_2024b_Jetson/1 - Experiment Logic/Phase #5: Hold Home/Desired Position RED ==
  Constant2 : Constant  Value=home_states_RED
  Target Array : Outport
  wires:
  Constant2/1 -> Target Array/1

== system Template_v4_1_0_2024b_Jetson/2 - Guidance/Custom PPL (ARM)/Desired Position ==
  Data Store Read : DataStoreRead  DataStoreName=ARM_Desired_States  IndexOptions=Index vector (dialog)  Indices=1  OutputSizes=1
  Position Array : Outport
  wires:
  Data Store Read/1 -> Position Array/1

== system Template_v4_1_0_2024b_Jetson/2 - Guidance/Custom PPL (BLACK)/Desired Position ==
  BLACK_Px : DataStoreRead  DataStoreName=BLACK_Desired_States  IndexOptions=Index vector (dialog)  Indices=1  OutputSizes=1
  Position Array : Outport
  wires:
  BLACK_Px/1 -> Position Array/1

== system Template_v4_1_0_2024b_Jetson/2 - Guidance/Custom PPL (BLUE)/Desired Position ==
  Data Store Read4 : DataStoreRead  DataStoreName=BLUE_Desired_States  IndexOptions=Index vector (dialog)  Indices=1  OutputSizes=1
  Position Array : Outport
  wires:
  Data Store Read4/1 -> Position Array/1

== system Template_v4_1_0_2024b_Jetson/2 - Guidance/Custom PPL (RED)/Desired Position ==
  RED_Px : DataStoreRead  DataStoreName=RED_Desired_States  IndexOptions=Index vector (dialog)  Indices=1  OutputSizes=1
  Position Array : Outport
  wires:
  RED_Px/1 -> Position Array/1

== system Template_v4_1_0_2024b_Jetson/2 - Guidance/Default APF PPL (BLACK)/Current Position RED ==
  Demux : Demux  Outputs=[3,6]
  RED_Px : DataStoreRead  DataStoreName=BLACK_Measured_States  IndexOptions=Index vector (dialog)  Indices=1  OutputSizes=1
  Terminator : Terminator
  Position Array : Outport
  wires:
  RED_Px/1 -> Demux/1
  Demux/1 -> Position Array/1
  Demux/2 -> Terminator/1

== system Template_v4_1_0_2024b_Jetson/2 - Guidance/Default APF PPL (BLACK)/Obstacles ==
  Current Position BLUE : Subsystem
  Current Position RED : Subsystem
  Matrix Concatenate : Concatenate  Mode=Multidimensional array
  Obstacle Positions : Outport
  wires:
  Current Position RED/1(Position Array) -> Matrix Concatenate/2
  Current Position BLUE/1(Position Array) -> Matrix Concatenate/1
  Matrix Concatenate/1 -> Obstacle Positions/1

== system Template_v4_1_0_2024b_Jetson/2 - Guidance/Default APF PPL (RED)/Current Position RED ==
  Demux : Demux  Outputs=[3,6]
  RED_Px : DataStoreRead  DataStoreName=RED_Measured_States  IndexOptions=Index vector (dialog)  Indices=1  OutputSizes=1
  Terminator : Terminator
  Position Array : Outport
  wires:
  RED_Px/1 -> Demux/1
  Demux/1 -> Position Array/1
  Demux/2 -> Terminator/1

== system Template_v4_1_0_2024b_Jetson/2 - Guidance/Default APF PPL (RED)/Obstacles ==
  Current Position BLACK : Subsystem
  Current Position BLUE : Subsystem
  Matrix Concatenate : Concatenate  Mode=Multidimensional array
  Obstacle Positions : Outport
  wires:
  Current Position BLACK/1(Position Array) -> Matrix Concatenate/2
  Current Position BLUE/1(Position Array) -> Matrix Concatenate/1
  Matrix Concatenate/1 -> Obstacle Positions/1

== system Template_v4_1_0_2024b_Jetson/2 - Guidance/Disable PPL (ARM)/Desired Position ==
  Data Store Read : DataStoreRead  DataStoreName=ARM_Desired_States  IndexOptions=Index vector (dialog)  Indices=1  OutputSizes=1
  Position Array : Outport
  wires:
  Data Store Read/1 -> Position Array/1

== system Template_v4_1_0_2024b_Jetson/2 - Guidance/Disable PPL (BLACK)/Desired Position ==
  BLACK_Px : DataStoreRead  DataStoreName=BLACK_Desired_States  IndexOptions=Index vector (dialog)  Indices=1  OutputSizes=1
  Position Array : Outport
  wires:
  BLACK_Px/1 -> Position Array/1

== system Template_v4_1_0_2024b_Jetson/2 - Guidance/Disable PPL (BLUE)/Desired Position ==
  Data Store Read4 : DataStoreRead  DataStoreName=BLUE_Desired_States  IndexOptions=Index vector (dialog)  Indices=1  OutputSizes=1
  Position Array : Outport
  wires:
  Data Store Read4/1 -> Position Array/1

== system Template_v4_1_0_2024b_Jetson/2 - Guidance/Disable PPL (RED)/Desired Position ==
  RED_Px : DataStoreRead  DataStoreName=RED_Desired_States  IndexOptions=Index vector (dialog)  Indices=1  OutputSizes=1
  Position Array : Outport
  wires:
  RED_Px/1 -> Position Array/1

== system Template_v4_1_0_2024b_Jetson/3 - Control/Default LQR Control (BLACK)/Calculate Error ==
  Unwrapped Angle : Inport
  Unwrapped Angle1 : Inport  Port=2
  Subtract3 : Sum  Inputs=-+
  Unwrap : dspsigops/Unwrap  tol=pi  InputProcessing=Columns as channels (frame based)  running=off
  Unwrap1 : dspsigops/Unwrap  tol=pi  InputProcessing=Columns as channels (frame based)  running=off
  Wrap : Subsystem
  Wrap1 : Subsystem
  Attitude Error : Outport
  wires:
  Unwrapped Angle1/1 -> Wrap1/1(Unwrapped Angle)
  Unwrap/1 -> Subtract3/1
  Unwrap1/1 -> Subtract3/2
  Wrap/1(Wrapped Angle) -> Unwrap/1
  Unwrapped Angle/1 -> Wrap/1(Unwrapped Angle)
  Wrap1/1(Wrapped Angle) -> Unwrap1/1
  Subtract3/1 -> Attitude Error/1

== system Template_v4_1_0_2024b_Jetson/3 - Control/Default LQR Control (BLUE)/Calculate Error ==
  Unwrapped Angle : Inport
  Unwrapped Angle1 : Inport  Port=2
  Subtract3 : Sum  Inputs=-+
  Unwrap : dspsigops/Unwrap  tol=pi  InputProcessing=Columns as channels (frame based)  running=off
  Unwrap1 : dspsigops/Unwrap  tol=pi  InputProcessing=Columns as channels (frame based)  running=off
  Wrap : Subsystem
  Wrap1 : Subsystem
  Attitude Error : Outport
  wires:
  Unwrapped Angle1/1 -> Wrap1/1(Unwrapped Angle)
  Unwrap/1 -> Subtract3/1
  Unwrap1/1 -> Subtract3/2
  Wrap/1(Wrapped Angle) -> Unwrap/1
  Unwrapped Angle/1 -> Wrap/1(Unwrapped Angle)
  Wrap1/1(Wrapped Angle) -> Unwrap1/1
  Subtract3/1 -> Attitude Error/1

== system Template_v4_1_0_2024b_Jetson/3 - Control/Default LQR Control (RED)/Calculate Error ==
  Unwrapped Angle : Inport
  Unwrapped Angle1 : Inport  Port=2
  Subtract3 : Sum  Inputs=-+
  Unwrap : dspsigops/Unwrap  tol=pi  InputProcessing=Columns as channels (frame based)  running=off
  Unwrap1 : dspsigops/Unwrap  tol=pi  InputProcessing=Columns as channels (frame based)  running=off
  Wrap : Subsystem
  Wrap1 : Subsystem
  Attitude Error : Outport
  wires:
  Unwrapped Angle1/1 -> Wrap1/1(Unwrapped Angle)
  Unwrap/1 -> Subtract3/1
  Unwrap1/1 -> Subtract3/2
  Wrap/1(Wrapped Angle) -> Unwrap/1
  Unwrapped Angle/1 -> Wrap/1(Unwrapped Angle)
  Wrap1/1(Wrapped Angle) -> Unwrap1/1
  Subtract3/1 -> Attitude Error/1

== system Template_v4_1_0_2024b_Jetson/3 - Control/Default PD (ARM)/Passthrough for Experiment ==
  q1_desired : Inport
  q2_desired : Inport  Port=2
  q3_desired : Inport  Port=3
  Action Port : ActionPort  ActionPortLabel=else
  q1_command : Outport
  q2_command : Outport  Port=2
  q3_command : Outport  Port=3
  wires:
  q3_desired/1 -> q3_command/1
  q1_desired/1 -> q1_command/1
  q2_desired/1 -> q2_command/1

== system Template_v4_1_0_2024b_Jetson/3 - Control/Default PD (ARM)/Simulated Position Controller ==
  q1_desired : Inport
  q2_desired : Inport  Port=2
  q3_desired : Inport  Port=3
  Action Port : ActionPort  ActionPortLabel=if(u1 == 1)
  Custom Discrete PD (Elbow) : Subsystem
  Custom Discrete PD (Shoulder) : Subsystem
  Custom Discrete PD (Wrist) : Subsystem
  Data Store Read2 : DataStoreRead  DataStoreName=ARM_Measured_States  IndexOptions=Index vector (dialog)  Indices=1  OutputSizes=1
  Demux : Demux  Outputs=[1,1,1,3]
  Saturation : Saturate  UpperLimit=Tz_lim_sharm  LowerLimit=-Tz_lim_sharm
  Saturation1 : Saturate  UpperLimit=Tz_lim_elarm  LowerLimit=-Tz_lim_elarm
  Saturation3 : Saturate  UpperLimit=Tz_lim_wrarm  LowerLimit=-Tz_lim_wrarm
  Subtract2 : Sum  Inputs=+-
  Subtract3 : Sum  Inputs=+-
  Subtract4 : Sum  Inputs=+-
  Terminator : Terminator
  q1_command : Outport
  q2_command : Outport  Port=2
  q3_command : Outport  Port=3
  wires:
  Saturation3/1 -> q3_command/1
  Subtract4/1 -> Custom Discrete PD (Wrist)/1(ey)
  Custom Discrete PD (Shoulder)/1(Fx) -> Saturation/1
  Custom Discrete PD (Elbow)/1(Fy) -> Saturation1/1
  Saturation/1 -> q1_command/1
  Subtract2/1 -> Custom Discrete PD (Shoulder)/1(ex)
  Saturation1/1 -> q2_command/1
  Custom Discrete PD (Wrist)/1(Fy) -> Saturation3/1
  Subtract3/1 -> Custom Discrete PD (Elbow)/1(ey)
  Demux/1 -> Subtract2/2
  Demux/2 -> Subtract3/2
  Demux/3 -> Subtract4/2
  q1_desired/1 -> Subtract2/1
  q2_desired/1 -> Subtract3/1
  q3_desired/1 -> Subtract4/1
  Data Store Read2/1 -> Demux/1
  Demux/4 -> Terminator/1

== system Template_v4_1_0_2024b_Jetson/3 - Control/Default PD Control (BLACK)/Calculate Error ==
  Unwrapped Angle : Inport
  Unwrapped Angle1 : Inport  Port=2
  Subtract3 : Sum  Inputs=-+
  Unwrap : dspsigops/Unwrap  tol=pi  InputProcessing=Columns as channels (frame based)  running=off
  Unwrap1 : dspsigops/Unwrap  tol=pi  InputProcessing=Columns as channels (frame based)  running=off
  Wrap : Subsystem
  Wrap1 : Subsystem
  Attitude Error : Outport
  wires:
  Unwrapped Angle1/1 -> Wrap1/1(Unwrapped Angle)
  Unwrap/1 -> Subtract3/1
  Unwrap1/1 -> Subtract3/2
  Wrap/1(Wrapped Angle) -> Unwrap/1
  Unwrapped Angle/1 -> Wrap/1(Unwrapped Angle)
  Wrap1/1(Wrapped Angle) -> Unwrap1/1
  Subtract3/1 -> Attitude Error/1

== system Template_v4_1_0_2024b_Jetson/3 - Control/Default PD Control (BLUE)/Calculate Error ==
  Unwrapped Angle : Inport
  Unwrapped Angle1 : Inport  Port=2
  Subtract3 : Sum  Inputs=-+
  Unwrap : dspsigops/Unwrap  tol=pi  InputProcessing=Columns as channels (frame based)  running=off
  Unwrap1 : dspsigops/Unwrap  tol=pi  InputProcessing=Columns as channels (frame based)  running=off
  Wrap : Subsystem
  Wrap1 : Subsystem
  Attitude Error : Outport
  wires:
  Unwrapped Angle1/1 -> Wrap1/1(Unwrapped Angle)
  Unwrap/1 -> Subtract3/1
  Unwrap1/1 -> Subtract3/2
  Wrap/1(Wrapped Angle) -> Unwrap/1
  Unwrapped Angle/1 -> Wrap/1(Unwrapped Angle)
  Wrap1/1(Wrapped Angle) -> Unwrap1/1
  Subtract3/1 -> Attitude Error/1

== system Template_v4_1_0_2024b_Jetson/3 - Control/Default PD Control (RED)/Calculate Error ==
  Unwrapped Angle : Inport
  Unwrapped Angle1 : Inport  Port=2
  Subtract3 : Sum  Inputs=-+
  Unwrap : dspsigops/Unwrap  tol=pi  InputProcessing=Columns as channels (frame based)  running=off
  Unwrap1 : dspsigops/Unwrap  tol=pi  InputProcessing=Columns as channels (frame based)  running=off
  Wrap : Subsystem
  Wrap1 : Subsystem
  Attitude Error : Outport
  wires:
  Unwrapped Angle1/1 -> Wrap1/1(Unwrapped Angle)
  Unwrap/1 -> Subtract3/1
  Unwrap1/1 -> Subtract3/2
  Wrap/1(Wrapped Angle) -> Unwrap/1
  Unwrapped Angle/1 -> Wrap/1(Unwrapped Angle)
  Wrap1/1(Wrapped Angle) -> Unwrap1/1
  Subtract3/1 -> Attitude Error/1

== system Template_v4_1_0_2024b_Jetson/PhaseSpace Camera Code/Use Hardware to Obtain States/Receive and Process Phasespace Data ==
  "Adjust Time " : Subsystem
  Check for Sychronization : Subsystem
  Clock : Clock
  Demux2 : Demux  Outputs=[1,18]
  Mux : Mux  Inputs=2
  Receive PhaseSpace Data : nvidiaSharedBlocks/UDP Receive  localURL='0.0.0.0'  localPort=31534  remoteURL='0.0.0.0'  remotePort=-1  recvBufferSize=8192  signalDatatype=double  dims=19  isVarSize=off  showBlockingTime=off  blockingTime=0  sampletime=-1  blockPlatform=NVIDIA
  Reshape : Reshape  OutputDimensionality=Customize  OutputDimensions=[19,1]
  Terminator : Terminator
  PhaseSpace Data : Outport
  PhaseSpace Clock : Outport  Port=2
  wires:
  Check for Sychronization/1(StartClock) -> "Adjust Time "/1(ClockStart)
  Reshape/1 -> Demux2/1
  "Adjust Time "/1(ClockAdjusted) -> Mux/1
  Demux2/2 -> Mux/2
  Mux/1 -> PhaseSpace Data/1
  Receive PhaseSpace Data/2 -> Terminator/1
  Receive PhaseSpace Data/1 -> Reshape/1
  Clock/1 -> "Adjust Time "/2(ClockRaw)
  Demux2/1 -> PhaseSpace Clock/1

== system Template_v4_1_0_2024b_Jetson/PhaseSpace Camera Code/Use Hardware to Obtain States/Store BLACK Data ==
  note: Store BLACK Positions and Velocities
  BLACK Data : Inport
  BLACK Velocities : Inport  Port=2
  PS Clock : Inport  Port=3
  Calculate True Time Step : Subsystem
      settings: PortSchema="{\"entries\":[{\"content\":{\"sides\":[{\"content\":{\"connectorIds\":[\"In1\"]},\"type\":\"ConnectorPlacement.EquallySpacedRectSide\",\"uuid\":\"62932c5c-f2a7-44c8-96b4-4a75bab3a126\"},{\"content\":{\"connectorIds\":[\"Out1\"],\"side\":\"RIGHT\"},\"type\":\"ConnectorPlacement.EquallySpacedRectSide\",\"uuid\":\"82b3b717-2171-4047-b0df-3cd41cf9dfc7\"},{\"content\":{\"side\":\"TOP\"},\"type\":\"ConnectorPlacement.EquallySpacedRectSide\",\"uuid\":\"a142272a-a0ff-4882-8a2d-4633b3c7e02f\"},{\"content\":{\"connectorIds\":[\"In2\"],\"side\":\"BOTTOM\"},\"type\":\"ConnectorPlacement.EquallySpacedRectSide\",\"uuid\":\"b1e1ff4c-66d6-488f-92fb-77f76780833b\"}]},\"type\":\"ConnectorPlacement.EquallySpacedConnector\",\"uuid\":\"98c51868-8a10-4b52-aae4-56f6042c65c4\"}],\"packageUris\":[\"http://schema.mathworks.com/mf0/Connector/R2020b\"],\"version\":\"1.0\"}"
  Convert BLACKVX from [mm] to [m] : Gain  Gain=1/1000
  Convert BLACKVY from [mm] to [m] : Gain  Gain=1/1000
  Convert BLAX from [mm] to [m] : Gain  Gain=1/1000
  Convert BLAY from [mm] to [m] : Gain  Gain=1/1000
  Demux : Demux  Outputs=3
  Demux2 : Demux  Outputs=3
  Demux3 : Demux  Outputs=3
  Mux{1..4} (4 alike) : Mux  Inputs=3
  RED_Px7 : DataStoreWrite  DataStoreName=BLACK_Measured_States  IndexOptions=Index vector (dialog)  Indices=1  OutputSizes=1
  Reshape : Reshape  OutputDimensionality=Column vector (2-D)
  Subsystem1 : Subsystem
  Subsystem2 : Subsystem
  Wrap : Subsystem
  wires:
  Demux3/1 -> Convert BLAX from [mm] to [m]/1
  Demux3/2 -> Convert BLAY from [mm] to [m]/1
  BLACK Data/1 -> Demux3/1
  Demux/3 -> Wrap/1(Unwrapped Angle)
  Reshape/1 -> Subsystem1/2(y)
  Demux/1 -> Mux1/1
  Convert BLAY from [mm] to [m]/1 -> Mux3/2
  Calculate True Time Step/1(dt_out) -> Subsystem2/1(dt), Subsystem1/1(dt)
  Mux3/1 -> Subsystem2/2(y), Demux/1, Calculate True Time Step/2(Data)
  Wrap/1(Wrapped Angle) -> Mux1/3
  Convert BLAX from [mm] to [m]/1 -> Mux3/1
  Mux2/1 -> RED_Px7/1
  Demux/2 -> Mux1/2
  Subsystem2/1(dy/dt) -> Reshape/1
  PS Clock/1 -> Calculate True Time Step/1(Time)
  Demux3/3 -> Mux3/3
  Mux1/1 -> Mux2/1
  Subsystem1/1(dy/dt) -> Mux2/3
  BLACK Velocities/1 -> Demux2/1
  Demux2/3 -> Mux4/3
  Convert BLACKVX from [mm] to [m]/1 -> Mux4/1
  Convert BLACKVY from [mm] to [m]/1 -> Mux4/2
  Mux4/1 -> Mux2/2
  Demux2/2 -> Convert BLACKVY from [mm] to [m]/1
  Demux2/1 -> Convert BLACKVX from [mm] to [m]/1
